simulink library "sltestProjectorCtrlLibrary"  (R2016a)
settings: Solver=ode45  StartTime=0.0  StopTime=10.0  RelTol=1e-3
settings Model: Creator=The MathWorks, Inc.  LastModifiedBy=The MathWorks, Inc.
settings DataIOCC: LimitDataPoints=on  SaveFormat=Array
settings DebuggingCC: SolverPrmCheckMsg=warning  AllowSymbolicDim=off
settings ModelReferenceCC: PropagateSignalLabelsOutOfModel=off
settings ConfigComp: CovModelRefEnable=Off  CovSFcnEnable=off

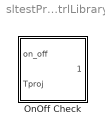
== system sltestProjectorCtrlLibrary ==
  OnOff Check : Subsystem  TreatAsAtomicUnit=on

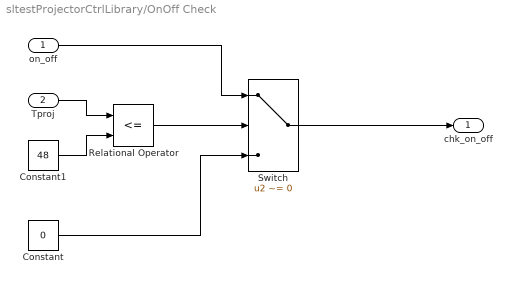
== system sltestProjectorCtrlLibrary/OnOff Check ==
  on_off : Inport  OutDataTypeStr=boolean
  Tproj : Inport  Port=2  OutMin=[0]  OutDataTypeStr=single
  Constant : Constant  Value=0  OutDataTypeStr=boolean
  Constant1 : Constant  Value=48  OutDataTypeStr=single
  Relational Operator : RelationalOperator  Operator=<=  OutDataTypeStr=boolean
  Switch : Switch  Criteria=u2 ~= 0
  chk_on_off : Outport
  wires:
  on_off/1 -> Switch/1
  Constant1/1 -> Relational Operator/2
  Tproj/1 -> Relational Operator/1
  Relational Operator/1 -> Switch/2
  Constant/1 -> Switch/3
  Switch/1 -> chk_on_off/1
